simulink model "dyn_zlin_mod_ciagly"  (R2014b)
settings: Solver=ode45  StartTime=0.0  StopTime=100  RelTol=1e-3
values from neighbouring files (symbols this model uses):
  a1 = 0.39    [dane_poczatkowe.mat]
  a2 = 0.45    [dane_poczatkowe.mat]
  a3 = -2.91    [dane_poczatkowe.mat]
  a4 = 0.25    [dane_poczatkowe.mat]
  K = 3.5    [dane_poczatkowe.mat]
  T1 = 5    [dane_poczatkowe.mat]
  T2 = 9    [dane_poczatkowe.mat]
undefined symbols (not defined in the file or in its folder): U, x1, x2
settings Model: Creator=Konrad  LastModifiedBy=Konrad

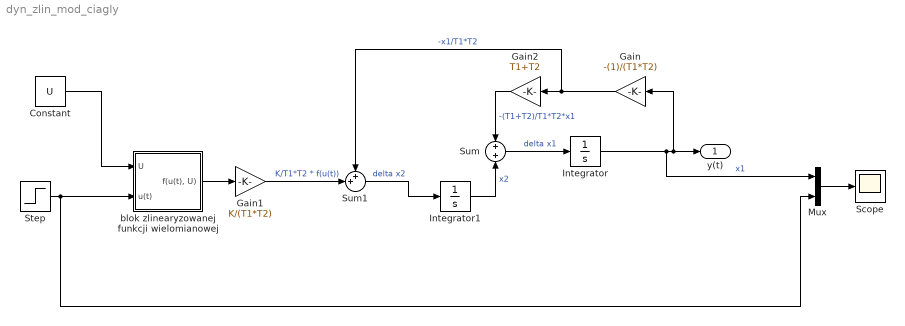
== system dyn_zlin_mod_ciagly ==
  Constant : Constant  Value=U
  Gain : Gain  Gain=-(1)/(T1*T2)
  Gain1 : Gain  Gain=K/(T1*T2)
  Gain2 : Gain  Gain=T1+T2
  Integrator : Integrator  InitialCondition=x1  ContinuousStateAttributes='x1'
  Integrator1 : Integrator  InitialCondition=x2  ContinuousStateAttributes='x2'
  Mux : Mux  Inputs=2
  Scope : Scope
  Step : Step  SampleTime=0
  Sum : Sum
  Sum1 : Sum  Inputs=++|
  blok zlinearyzowanej funkcji wielomianowej : Subsystem
  y(t) : Outport
  wires:
  Integrator/1 -> Mux/1, Gain/1, y(t)/1  "x1"
  Sum/1 -> Integrator/1  "delta x1"
  Integrator1/1 -> Sum/2  "x2"
  Gain/1 -> Sum1/1, Gain2/1  "-x1/T1*T2"
  Gain2/1 -> Sum/1  "-(T1+T2)/T1*T2*x1"
  Sum1/1 -> Integrator1/1  "delta x2"
  Gain1/1 -> Sum1/2  "K/T1*T2 * f(u(t))"
  blok zlinearyzowanej funkcji wielomianowej/1("f(u(t), U)") -> Gain1/1
  Step/1 -> blok zlinearyzowanej funkcji wielomianowej/2(u(t)), Mux/2
  Mux/1 -> Scope/1
  Constant/1 -> blok zlinearyzowanej funkcji wielomianowej/1(U)

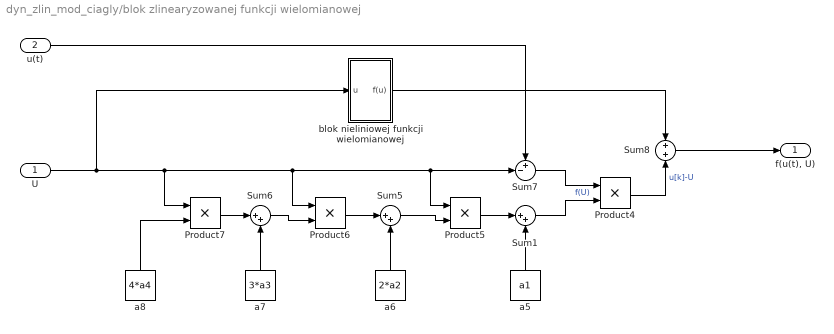
== system dyn_zlin_mod_ciagly/blok zlinearyzowanej funkcji wielomianowej ==
  U : Inport
  u(t) : Inport  Port=2
  Product{4..7} (4 alike) : Product
  Sum1 : Sum  Inputs=|++
  Sum5 : Sum  Inputs=|++
  Sum6 : Sum  Inputs=|++
  Sum7 : Sum  Inputs=+-|
  Sum8 : Sum
  a5 : Constant  Value=a1
  a6 : Constant  Value=2*a2
  a7 : Constant  Value=3*a3
  a8 : Constant  Value=4*a4
  blok nieliniowej funkcji wielomianowej : Subsystem
  "f(u(t), U)" : Outport
  wires:
  U/1 -> blok nieliniowej funkcji wielomianowej/1(u), Product5/1, Sum7/2, Product6/1, Product7/1
  Product5/1 -> Sum1/1
  Product6/1 -> Sum5/1
  Product7/1 -> Sum6/1
  a5/1 -> Sum1/2
  a6/1 -> Sum5/2
  Sum5/1 -> Product5/2
  a7/1 -> Sum6/2
  Sum6/1 -> Product6/2
  a8/1 -> Product7/2
  Sum1/1 -> Product4/2  "f(U)"
  Sum7/1 -> Product4/1
  u(t)/1 -> Sum7/1
  Product4/1 -> Sum8/2  "u[k]-U"
  Sum8/1 -> "f(u(t), U)"/1
  blok nieliniowej funkcji wielomianowej/1(f(u)) -> Sum8/1

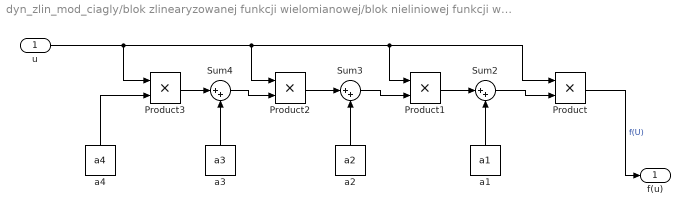
== system dyn_zlin_mod_ciagly/blok zlinearyzowanej funkcji wielomianowej/blok nieliniowej funkcji wielomianowej ==
  u : Inport
  Product{,1..3} (4 alike) : Product
  Sum2 : Sum  Inputs=|++
  Sum3 : Sum  Inputs=|++
  Sum4 : Sum  Inputs=|++
  a1 : Constant  Value=a1
  a2 : Constant  Value=a2
  a3 : Constant  Value=a3
  a4 : Constant  Value=a4
  f(u) : Outport
  wires:
  u/1 -> Product/1, Product1/1, Product2/1, Product3/1
  Product2/1 -> Sum3/1
  Sum2/1 -> Product/2
  Product/1 -> f(u)/1  "f(U)"
  Product3/1 -> Sum4/1
  a1/1 -> Sum2/2
  a2/1 -> Sum3/2
  Sum3/1 -> Product1/2
  Sum4/1 -> Product2/2
  a3/1 -> Sum4/2
  a4/1 -> Product3/2
  Product1/1 -> Sum2/1
